simulink model "Control_Simulink"  (R2015a)
settings: Solver=ode3  StartTime=0  StopTime=tf  FixedStep=t_step  RelTol=1e-3
values from neighbouring files (symbols this model uses):
  A = [ -1/(Cf*(Rl+RCf)),          Rl/(Cf*(Rl+RCf)) ... (first row only)    [Controller.m]    (also in Controller_ID.m; Controller_ID_Noise.m; Controller_MOD_Hard.m; Controller_MOD_Soft.m)
  Ad = sysd.a    [Controller.m]    (also in Controller_ID.m = [0.997804369618173, 0.014625348088769; Controller_ID_Noise.m = [0.997804369618173, 0.014625348088769; Controller_MOD_Hard.m = [0.997804369618173, 0.014625348088769; Controller_MOD_Soft.m = [0.997804369618173, 0.014625348088769)
  B = [0;  Vi/(N*Lf)]    [Controller.m]    (also in Controller_ID.m; Controller_ID_Noise.m; Controller_MOD_Hard.m; Controller_MOD_Soft.m)
  Bd = sysd.b    [Controller.m]    (also in Controller_ID.m = [0.087557083891431; 11.941525420783089]; Controller_ID_Noise.m = [0.087557083891431; 11.941525420783089]; Controller_MOD_Hard.m = [0.087557083891431; 11.941525420783089]; Controller_MOD_Soft.m = [0.087557083891431; 11.941525420783089])
  C = [Rl/(Rl+RCf),  Rl*RCf/(Rl+RCf)]    [Controller.m]    (also in Controller_ID.m; Controller_ID_Noise.m; Controller_MOD_Hard.m; Controller_MOD_Soft.m)
  Cd = sysd.c    [Controller.m]    (also in Controller_ID.m = [0.995766824623838, 0.028197671115147]; Controller_ID_Noise.m = [0.995766824623838, 0.028197671115147]; Controller_MOD_Hard.m = [0.995766824623838, 0.028197671115147]; Controller_MOD_Soft.m = [0.995766824623838, 0.028197671115147])
  D = 0    [Controller.m]    (also in Controller_ID.m; Controller_ID_Noise.m; Controller_MOD_Hard.m; Controller_MOD_Soft.m)
  Dmax = 0.366357    [Bridge_Bulk.m]    (also in Controller.m = 0.45; Controller_ID.m = 0.45; Controller_ID_Noise.m = 0.45; Controller_MOD_Hard.m = 0.45)
  G = 1 / (30 / Sat_max)    (= 0.166666666667)    [Controller.m]    (also in Controller_ID.m; Controller_ID_Noise.m; Controller_MOD_Hard.m; Controller_MOD_Soft.m)
  K = dlqr(alpha*Ad_aug, alpha*Bd_aug, Q1, Q2)    [Controller.m]    (also in Controller_ID.m = [0.033293762099687, 0.032463881530606,      0.00023052612695; Controller_ID_Noise.m = [0.033293762099687, 0.032463881530606,      0.00023052612695; Controller_MOD_Hard.m = [0.033293762099687, 0.032463881530606,      0.00023052612695; Controller_MOD_Soft.m = [0.033293762099687, 0.032463881530606,      0.00023052612695)
  Le = place(Ad', Cd', Pz_obs)'    [Controller.m]    (also in Controller_ID.m = [0.349035208102762; 8.644382966325479]; Controller_ID_Noise.m = [0.349035208102762; 8.644382966325479]; Controller_MOD_Hard.m = [0.349035208102762; 8.644382966325479]; Controller_MOD_Soft.m = [0.349035208102762; 8.644382966325479])
  Sat_max = 5    [Controller.m]    (also in Controller_ID.m; Controller_ID_Noise.m; Controller_MOD_Hard.m; Controller_MOD_Soft.m)
  Sat_min = 0    [Controller.m]    (also in Controller_ID.m; Controller_ID_Noise.m; Controller_MOD_Hard.m; Controller_MOD_Soft.m)
  t_step = Ts / 10    (= 1e-06)    [Controller.m]    (also in Controller_ID.m; Controller_ID_Noise.m; Controller_MOD_Hard.m; Controller_MOD_Soft.m)
  Ts = 1e-5    (= 1e-05)    [Controller.m]    (also in Controller_ID.m; Controller_ID_Noise.m; Controller_MOD_Hard.m; Controller_MOD_Soft.m)
  var_v = (0.01)^2    (= 0.0001)    [Controller.m]    (also in Controller_ID.m = 1e-08; Controller_ID_Noise.m; Controller_MOD_Hard.m; Controller_MOD_Soft.m)
  var_xd = var_v    (= 0.0001)    [Controller.m]    (also in Controller_ID.m = 1e-08; Controller_ID_Noise.m; Controller_MOD_Hard.m; Controller_MOD_Soft.m)
libraries: simulink x1
settings Model: Creator=Marcelo  LastModifiedBy=Marcelo
settings SolverCC: AutoInsertRateTranBlk=on

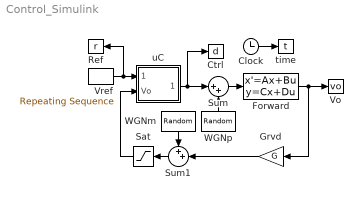
== system Control_Simulink ==
  Clock : Clock
  Ctrl : ToWorkspace  VariableName=d  SampleTime=-1
  Forward : StateSpace  A=A  B=B  C=C  D=D  X0=[0;0]
  Grvd : Gain  Gain=G
  Ref : ToWorkspace  VariableName=r  SampleTime=-1
  Sat : Saturate  UpperLimit=Sat_max  LowerLimit=Sat_min
  Sum : Sum  Inputs=|++
  Sum1 : Sum  Inputs=++|
  Vo : ToWorkspace  VariableName=vo  SampleTime=-1
  Vref : simulink/Sources/Repeating Sequence  rep_seq_t=[0, 0.02, 0.021, 0.04, 0.041, 0.06, 0.061]  rep_seq_y=[25, 25, 5, 5, 15, 15, 15]
  WGNm : RandomNumber  Variance=var_v  Seed=2  SampleTime=t_step
  WGNp : RandomNumber  Variance=var_xd  SampleTime=t_step
  time : ToWorkspace  VariableName=t  SampleTime=-1
  uC : Subsystem
  wires:
  Clock/1 -> time/1
  Sum/1 -> Forward/1
  Sum1/1 -> Sat/1
  Grvd/1 -> Sum1/2
  Forward/1 -> Grvd/1, Vo/1
  uC/1(Ctrl) -> Ctrl/1, Sum/1
  Vref/1 -> Ref/1, uC/1(Ref)
  Sat/1 -> uC/2(Vo)
  WGNm/1 -> Sum1/1
  WGNp/1 -> Sum/2

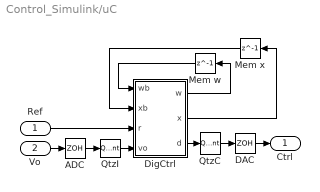
== system Control_Simulink/uC ==
  Ref : Inport
  Vo : Inport  Port=2
  ADC : ZeroOrderHold  SampleTime=Ts
  DAC : ZeroOrderHold  SampleTime=Ts
  DigCtrl : MATLAB Function  TreatAsAtomicUnit=on
  Mem w : Delay  DelayLength=1  InitialCondition=0  SampleTime=Ts
  Mem x : Delay  DelayLength=1  InitialCondition=[0;0]  SampleTime=Ts
  QtzC : Quantizer  QuantizationInterval=qtz_ctr  LinearizeAsGain=off
  QtzI : Quantizer  QuantizationInterval=qtz_in  LinearizeAsGain=off
  Ctrl : Outport
  wires:
  DigCtrl/1(w) -> Mem w/1
  Mem w/1 -> DigCtrl/1(wb)
  DigCtrl/2(x) -> Mem x/1
  Mem x/1 -> DigCtrl/2(xb)
  ADC/1 -> QtzI/1
  QtzI/1 -> DigCtrl/4(vo)
  Ref/1 -> DigCtrl/3(r)
  DigCtrl/3(d) -> QtzC/1
  QtzC/1 -> DAC/1
  DAC/1 -> Ctrl/1
  Vo/1 -> ADC/1

== matlab function Control_Simulink/uC/DigCtrl ==
  data: wb input; xb input; w output; x output; r input; vo input; d output; Ad parameter; Bd parameter; K parameter; Le parameter; Cd parameter; Dmax parameter
function [w, x, d] = fcn(wb, xb, r, vo, Ad, ...
    Bd, K, Le, Cd, Dmax)
% Plant output value correction
y = 6 * vo;
% Integral action
w = wb + y - r;
% Current Estimator - State update
x_LQG = xb + Le * (y - Cd*xb);
% Control effort
d = - K * [x_LQG; w];
% PWM saturation
if d > Dmax
    d = Dmax;
elseif d < 0
    d = 0;
end
% Current Estimator - State extrapolation
x = Ad*x_LQG + Bd*d;
